simulink model "Obiekt_inercyjny_II_rzedu"  (R2024b)
settings: Solver=ode4  StartTime=0.0  StopTime=20  FixedStep=0.01  RelTol=1e-3
model workspace (MAT data in the model file):
  A = [0  1; -0.428571428571  0]
  B = [0; 1]
  C = [1  0; 0  1]
  D = [0; 0]
  F = 1
  k = 6
  m = 14
  vx0 = [0.1; 0]
  x0 = 0.1
settings Model: Creator=mati  LastModifiedBy=mati

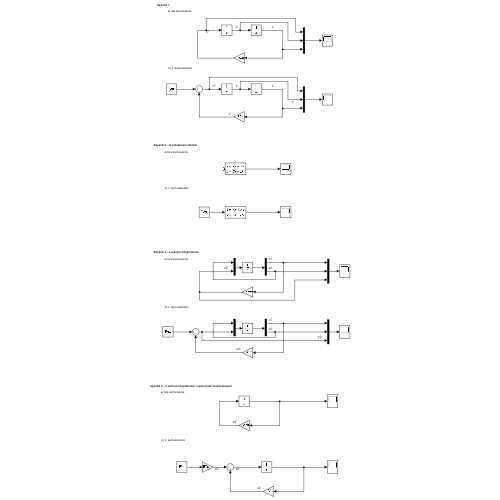
[thumbnail: Simulink's stored preview of the top-level diagram]
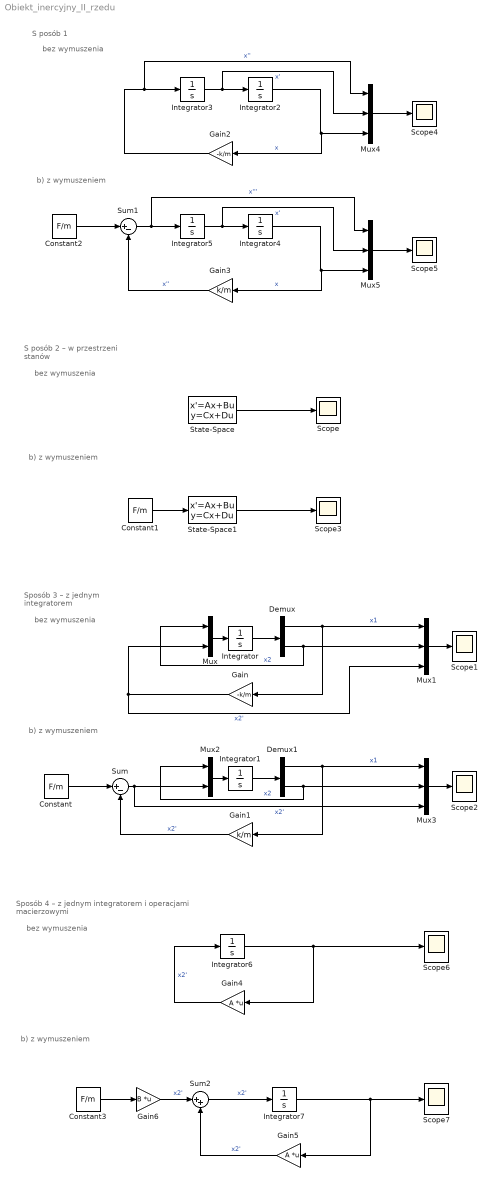
== system Obiekt_inercyjny_II_rzedu ==
  note: bez wymuszenia
  note: Sposób 3 – z jednym integratorem
  note: b) z wymuszeniem
  note: bez wymuszenia
  note: S posób 2 – w przestrzeni stanów
  note: b) z wymuszeniem
  note: S posób 1
  note: bez wymuszenia
  note: b) z wymuszeniem
  note: bez wymuszenia
  note: b) z wymuszeniem
  note: Sposób 4 – z jednym integratorem i operacjami macierzowymi
  Constant{,1..3} (4 alike) : Constant  Value=F/m
  Demux : Demux  Outputs=2
  Demux1 : Demux  Outputs=2
  Gain : Gain  Gain=-k/m
  Gain1 : Gain  Gain=k/m
  Gain2 : Gain  Gain=-k/m
  Gain3 : Gain  Gain=k/m
  Gain4 : Gain  Gain=A  Multiplication=Matrix(K*u)
  Gain5 : Gain  Gain=A  Multiplication=Matrix(K*u)
  Gain6 : Gain  Gain=B  Multiplication=Matrix(K*u)
  Integrator : Integrator  InitialCondition=vx0
  Integrator1 : Integrator  InitialCondition=vx0
  Integrator2 : Integrator  InitialCondition=x0
  Integrator3 : Integrator
  Integrator4 : Integrator  InitialCondition=x0
  Integrator5 : Integrator
  Integrator6 : Integrator  InitialCondition=[x0; 0]
  Integrator7 : Integrator  InitialCondition=vx0
  Mux : Mux  Inputs=2
  Mux{1,3..5} (4 alike) : Mux  Inputs=3
  Mux2 : Mux  Inputs=2
  Scope{,1..7} (8 alike) : Scope
  State-Space : StateSpace  A=A  B=[0;0]  C=C  D=D  InitialCondition=vx0
  State-Space1 : StateSpace  A=A  B=B  C=C  D=D  InitialCondition=vx0
  Sum : Sum  Inputs=|+-
  Sum1 : Sum  Inputs=|+-
  Sum2 : Sum  Inputs=|++
  wires:
  Mux/1 -> Integrator/1
  Integrator/1 -> Demux/1
  Demux/2 -> Mux/1, Mux1/2  "x2"
  Gain/1 -> Mux/2, Mux1/3  "x2'"
  Demux/1 -> Gain/1, Mux1/1  "x1"
  Mux1/1 -> Scope1/1
  Mux3/1 -> Scope2/1
  Demux1/2 -> Mux2/1, Mux3/2  "x2"
  Integrator1/1 -> Demux1/1
  Mux2/1 -> Integrator1/1
  Demux1/1 -> Gain1/1, Mux3/1  "x1"
  Constant/1 -> Sum/1
  Sum/1 -> Mux3/3, Mux2/2  "x2'"
  Gain1/1 -> Sum/2  "x2'"
  State-Space/1 -> Scope/1
  State-Space1/1 -> Scope3/1
  Constant1/1 -> State-Space1/1
  Mux4/1 -> Scope4/1
  Integrator3/1 -> Mux4/2, Integrator2/1  "x'"
  Integrator2/1 -> Gain2/1, Mux4/3  "x"
  Gain2/1 -> Mux4/1, Integrator3/1  "x''"
  Integrator4/1 -> Gain3/1, Mux5/3  "x"
  Mux5/1 -> Scope5/1
  Integrator5/1 -> Mux5/2, Integrator4/1  "x'"
  Sum1/1 -> Mux5/1, Integrator5/1  "x'''"
  Gain3/1 -> Sum1/2  "x''"
  Constant2/1 -> Sum1/1
  Integrator6/1 -> Scope6/1, Gain4/1
  Gain4/1 -> Integrator6/1  "x2'"
  Integrator7/1 -> Scope7/1, Gain5/1
  Constant3/1 -> Gain6/1
  Gain6/1 -> Sum2/1  "x2'"
  Sum2/1 -> Integrator7/1  "x2'"
  Gain5/1 -> Sum2/2  "x2'"
